simulink model "my_dom_state_space"  (R2018a)
settings: Solver=VariableStepAuto  StartTime=0.0  StopTime=10000  RelTol=1e-3
values from neighbouring files (symbols this model uses):
  A = [ -(a+K_1+K_w)/C_vw,    K_1/C_vw ... (first row only)    [leveled_NL.m]    (also in leveled_state_space.m = [ -(c_p*ro_p*f_p1+K_1+K_w)/C_vw,    K_1/C_vw; leveled_transmitancja.m; my_dom.m = [(T_wewN-T_pN), (T_wewN-T_zewN); my_dom_state_space_script.m)
  B = [ c_p*ro_p*f_pN/C_vw, K_w/C_vw ... (first row only)    [leveled_NL.m]    (also in leveled_state_space.m = [ c_p*ro_p*f_p1/C_vw, K_w/C_vw; leveled_transmitancja.m; my_dom.m = [a*(T_zN-T_wewN); 0]; my_dom_state_space_script.m)
  C = [1,0 ... (first row only)    [leveled_NL.m]    (also in leveled_state_space.m; leveled_transmitancja.m; my_dom_state_space_script.m; my_dom_trans_script.m)
  D = [0,0 ... (first row only)    [leveled_NL.m]    (also in leveled_state_space.m; leveled_transmitancja.m; my_dom_state_space_script.m; my_dom_trans_script.m)
  d_T_z = 0    [leveled_NL.m]    (also in leveled_state_space.m; leveled_transmitancja.m; my_dom.m; my_dom_state_space_script.m)
  d_T_zew = 0    [leveled_NL.m]    (also in leveled_state_space.m = 2; leveled_transmitancja.m = 2; my_dom.m; my_dom_state_space_script.m = 5)
  State_Space_Init = [T_wew0; T_p0]    [leveled_NL.m]    (also in leveled_state_space.m; leveled_transmitancja.m; my_dom_state_space_script.m)
  steptime = 1000    [leveled_NL.m]    (also in leveled_state_space.m; leveled_transmitancja.m; my_dom.m; my_dom_state_space_script.m)
  T_z1 = T_zN+8    (= 32)    [leveled_NL.m]    (also in leveled_state_space.m = 21; leveled_transmitancja.m = 21; my_dom.m = 29; my_dom_state_space_script.m = 24)
  T_zew1 = T_zewN-5    (= -6)    [leveled_NL.m]    (also in leveled_state_space.m = 4; leveled_transmitancja.m = 4; my_dom.m; my_dom_state_space_script.m = -1)
settings Model: Creator=johnb  LastModifiedBy=johnb

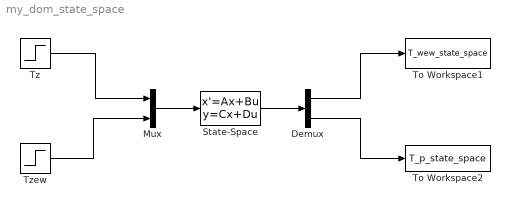
== system my_dom_state_space ==
  Demux : Demux  Outputs=2
  Mux : Mux  Inputs=2
  State-Space : StateSpace  A=A  B=B  C=C  D=D  InitialCondition=State_Space_Init
  To Workspace1 : ToWorkspace  VariableName=T_wew_state_space  SaveFormat=Timeseries  SampleTime=-1
  To Workspace2 : ToWorkspace  VariableName=T_p_state_space  SaveFormat=Timeseries  SampleTime=-1
  Tz : Step  Time=steptime  Before=T_z1  After=T_z1+d_T_z  SampleTime=0
  Tzew : Step  Time=steptime  Before=T_zew1  After=T_zew1+d_T_zew  SampleTime=0
  wires:
  Tz/1 -> Mux/1
  Mux/1 -> State-Space/1
  Demux/1 -> To Workspace1/1
  Demux/2 -> To Workspace2/1
  State-Space/1 -> Demux/1
  Tzew/1 -> Mux/2
